simulink model "gradfiltorg"  (R2014b)
settings: Solver=ode45  StartTime=0.0  StopTime=10.0  RelTol=1e-3
libraries: dspvision x2
settings Model: Creator=Shogo  LastModifiedBy=Shogo

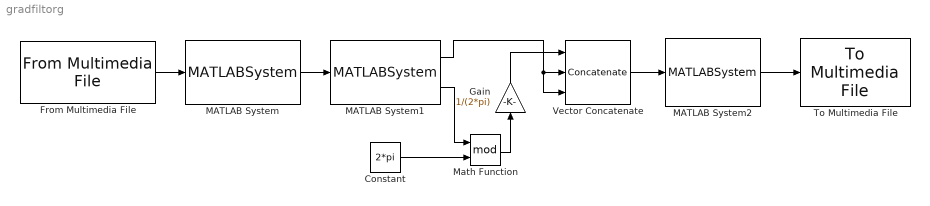
== system gradfiltorg ==
  Constant : Constant  Value=2*pi  OutDataTypeStr=single
  From Multimedia File : dspvision/From Multimedia File  inputFilename=vipmen.avi  loop=on  numPlays=inf  outputStreams=Video only  videoDataType=single  audioDataType=int16  inheritSampleTime=on  userDefinedSampleTime=1/30  noAudioOutput=off  isIntensityVideo=off  fourcc=RGB  colorVideoFormat=One multidimensional signal  outputEOF=off  dataOrg=Column-major  audioFrameSize=1024  computeAudioFrameSize=off  outSamplingMode=Sample based
  Gain : Gain  Gain=1/(2*pi)  OutDataTypeStr=single
  MATLAB System : MATLABSystem  System=embvision.Rgb2GraySystem
      mask Type: embvision.Rgb2GraySystem
      mask Display:
      | disp('RGB2GRAY');
      | port_label('input',1,'RGB');
      | port_label('output',1,'GRAY');
  MATLAB System1 : MATLABSystem  System=embvision.GradFiltSystem  Kernel=[ 1, 0, -1; 1, 0, -1; 1, 0, -1 ]
      mask Type: embvision.GradFiltSystem
      mask Display:
      | disp('GRAD_FILT');
      | port_label('input',1,'GRAY');
      | port_label('output',1,'MAG');
      | port_label('output',2,'ANG');
  MATLAB System2 : MATLABSystem  System=embvision.Hsv2RgbSystem
      mask Type: embvision.Hsv2RgbSystem
      mask Display:
      | disp('HSV2RGB');
      | port_label('input',1,'HSV');
      | port_label('output',1,'RGB');
  Math Function : Math  Operator=mod  OutputSignalType=real  SaturateOnIntegerOverflow=on
  To Multimedia File : dspvision/To Multimedia File  outputFilename=output.avi  streamSelection=Video only  videoCompressor=None (uncompressed)  audioCompressor=None (uncompressed)  imagePorts=One multidimensional signal  fileType=AVI  audioDatatype=Determine from input data type  fourcc=RGB  videoQuality=75  mj2000CompFactor=10
  Vector Concatenate : Concatenate  NumInputs=3  Mode=Multidimensional array  ConcatenateDimension=3
  wires:
  From Multimedia File/1 -> MATLAB System/1
  MATLAB System/1 -> MATLAB System1/1
  MATLAB System2/1 -> To Multimedia File/1
  Vector Concatenate/1 -> MATLAB System2/1
  MATLAB System1/1 -> Vector Concatenate/3, Vector Concatenate/2
  MATLAB System1/2 -> Math Function/1
  Math Function/1 -> Gain/1
  Gain/1 -> Vector Concatenate/1
  Constant/1 -> Math Function/2
